simulink model "full_state_smd_class"  (R2025a)
settings: Solver=VariableStepAuto  StartTime=0.0  StopTime=10  RelTol=1e-3
values from neighbouring files (symbols this model uses):
  A = [0 1 0 0 ; 0 -d/m m*g/M 0 ; 0 0 0 1; 0 -d/l*M (M+m)*g/(l*M) 0]    [CartPuller.m]    (also in Controller.m = [0 1 0 0; Ex12_4.m = [-5 1 0;0 -2 1;0 0 -1]; JacobCTP.m = [0 1 0 0; Observer_4state.m = [0 1; -k/m -c/m])
  B = [0 1/M 0 1/(M*l)]'    [CartPuller.m]    (also in Controller.m = [0;1/m1;0;0]; Ex12_4.m = [0;0;1]; Observer_4state.m = [0; 1/m]; full_order_observer_smd.m = [0 0 0 1/m2]')
  C = eye(4)    [Controller.m]    (also in Ex12_4.m = [-1 1 0]; Observer_4state.m = [1 0]; full_order_observer_smd.m = [1 0 0 0]; full_state_observer.m = [1 0 0 0])
  Ke = place(A_bb', A_ab', p_o)'    [Controller.m]    (also in Observer_4state.m = place(A', C', p_o)'; full_order_observer_smd.m = place(A',C',p)'; observer_E1.m = place(A', C', p_o); observer_sys.m = place(A', C', p_o)')
  x0 = [0;0;pi/3+0.1;0]    [CartPuller.m]    (also in CartPullerODE.m = [0;0;pi+0.1;0]; Controller.m = [1; 0; -1; 0]; JacobCTP.m = [0;0;pi+.1;0]; Observer_4state.m = [-2 0 -10 -1])
  x0_o = [2 1 -2 0.1]'    [full_order_observer_smd.m]    (also in simulink_observer.m)
settings Model: Creator=abhi  LastModifiedBy=abhi

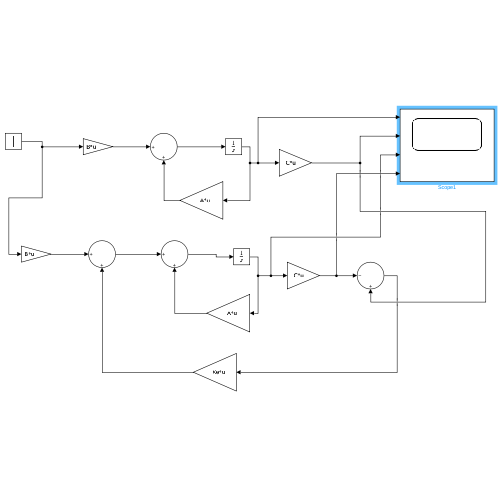
[thumbnail: Simulink's stored preview of the top-level diagram]
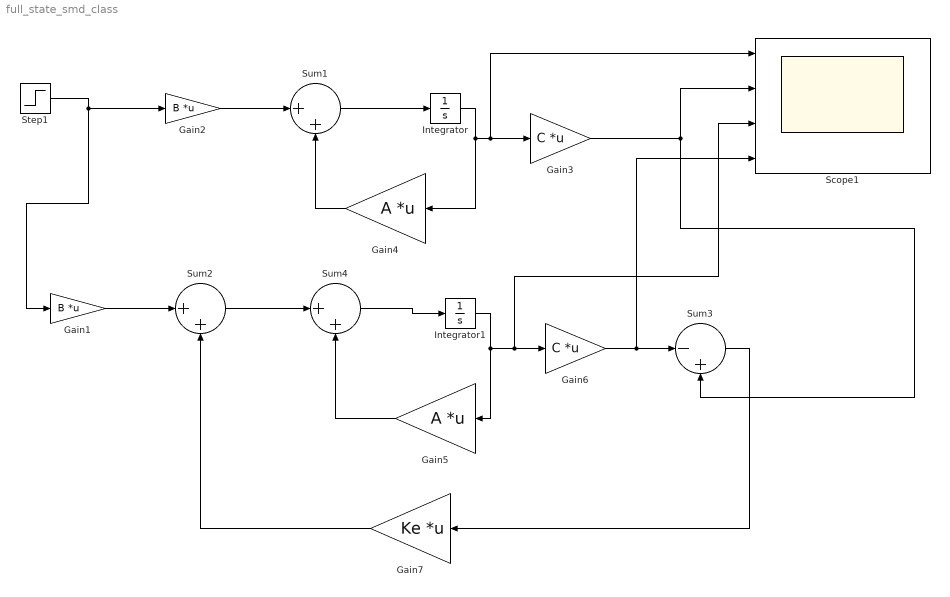
== system full_state_smd_class ==
  Gain1 : Gain  Gain=B  Multiplication=Matrix(K*u)
  Gain2 : Gain  Gain=B  Multiplication=Matrix(K*u)
  Gain3 : Gain  Gain=C  Multiplication=Matrix(K*u)
  Gain4 : Gain  Gain=A  Multiplication=Matrix(K*u)
  Gain5 : Gain  Gain=A  Multiplication=Matrix(K*u)
  Gain6 : Gain  Gain=C  Multiplication=Matrix(K*u)
  Gain7 : Gain  Gain=Ke  Multiplication=Matrix(K*u)
  Integrator : Integrator  InitialCondition=x0
  Integrator1 : Integrator  InitialCondition=x0_o
  Scope1 : Scope  NumInputPorts=4
      settings: SampleTime=1e-5  ActiveDisplayYMinimum=-0.0981688620159219  ActiveDisplayYMaximum=0.10097397600386415
  Step1 : Step  SampleTime=0
  Sum1 : Sum  Inputs=|++
  Sum2 : Sum  Inputs=|++
  Sum3 : Sum  Inputs=|-+
  Sum4 : Sum  Inputs=|++
  wires:
  Integrator/1 -> Scope1/1, Gain3/1, Gain4/1
  Gain4/1 -> Sum1/2
  Gain2/1 -> Sum1/1
  Step1/1 -> Gain1/1, Gain2/1
  Sum1/1 -> Integrator/1
  Gain3/1 -> Scope1/2, Sum3/2
  Integrator1/1 -> Scope1/3, Gain6/1, Gain5/1
  Gain5/1 -> Sum4/2
  Sum2/1 -> Sum4/1
  Sum4/1 -> Integrator1/1
  Gain6/1 -> Scope1/4, Sum3/1
  Sum3/1 -> Gain7/1
  Gain7/1 -> Sum2/2
  Gain1/1 -> Sum2/1
